simulink model "modelo_NL_con_modulador"  (R2018a)
settings: Solver=VariableStepAuto  StartTime=0.0  StopTime=30  MaxStep=1e-4  RelTol=1e-3
values from neighbouring files (symbols this model uses):
  alpha_Cu = 3.9e-3    (= 0.0039)    [proyecto_global_integrador.m]
  b_a = J_eq * n * w_pos    (= 0.0113019895361)    [proyecto_global_integrador.m]
  b_eq = b_m + b_l/r^2    (= 1.5e-05)    [proyecto_global_integrador.m]
  C_ts = 1.091    [proyecto_global_integrador.m]
  J_eq = J_m + J_l/r^2    (= 5.65099476805e-06)    [proyecto_global_integrador.m]
  k_sa = J_eq * n * w_pos^2    (= 9.04159162887)    [proyecto_global_integrador.m]
  k_sia = J_eq * w_pos^3    (= 2893.30932124)    [proyecto_global_integrador.m]
  Ke_theta = 2*polos_observador - b_eq/J_eq    (= 6397.34560009)    [proyecto_global_integrador.m]
  Ke_w = polos_observador^2 - Ke_theta * b_eq/J_eq    (= 10223018.8864)    [proyecto_global_integrador.m]
  L_d = 6.6e-3    (= 0.0066)    [proyecto_global_integrador.m]
  L_ls = 0.8e-3    (= 0.0008)    [proyecto_global_integrador.m]
  L_q = 5.8e-3    (= 0.0058)    [proyecto_global_integrador.m]
  lambda_m = 0.01546    [proyecto_global_integrador.m]
  P_p = 3    [proyecto_global_integrador.m]
  r = 314.3008    [proyecto_global_integrador.m]
  R_s = 1.02    [polos_choreo_no_se_puede_robar_mas_con_esto.m]    (also in proyecto_global_integrador.m)
  R_tsamb = 55    [proyecto_global_integrador.m]
  Rp_0 = 4    [proyecto_global_integrador.m]
  Rp_d = 33    [proyecto_global_integrador.m]
  Rp_q = 29    [proyecto_global_integrador.m]
  T_ambmax = 40    [proyecto_global_integrador.m]
libraries: simulink x4, peTransforms x2
settings Model: Creator=gabrielq  LastModifiedBy=wafle

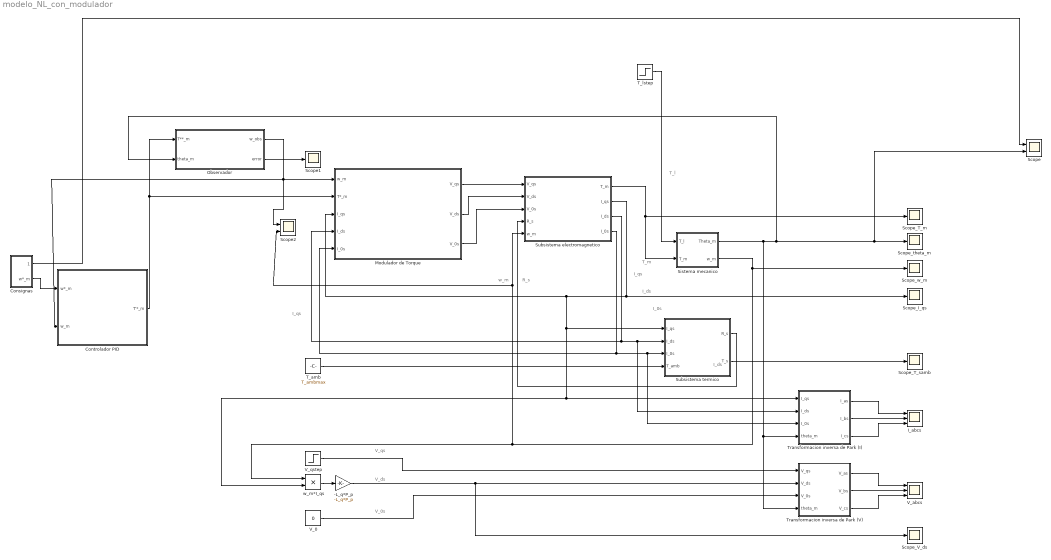
== system modelo_NL_con_modulador ==
  note: I_ds
  note: V_0s
  note: V_ds
  note: T_l
  note: V_qs
  note: T_m
  note: R_s
  note: I_0s
  note: I_ds
  note: I_qs
  note: I_qs
  note: w_m
  -L_q*P_p : Gain  Gain=-L_q*P_p
  Consignas : Subsystem
  Controlador PID : Subsystem
  I_abcs : Scope  NumInputPorts=3
  Modulador de Torque : Subsystem
  "Observador " : Subsystem
  Scope : Scope  NumInputPorts=2
  Scope1 : Scope
  Scope2 : Scope  NumInputPorts=2
  Scope_I_qs : Scope
  Scope_T_m : Scope
  Scope_T_samb : Scope
  Scope_V_ds : Scope
  Scope_theta_m : Scope
  Scope_w_m : Scope
  Sistema mecanico : Subsystem
  Subsistema electromagnetico : Subsystem
  Subsistema termico : Subsystem
  T_amb : Constant  Value=T_ambmax
  T_lstep : Step  Time=0.3  After=1.57  SampleTime=0
  Transformacion inversa de Park (I) : Subsystem
  Transformacion inversa de Park (V) : Subsystem
  V_0 : Constant  Value=0
  V_abcs : Scope  NumInputPorts=3
  V_qstep : Step  Time=0.1  After=19.596  SampleTime=0
  w_m*I_qs : Product
  wires:
  w_m*I_qs/1 -> -L_q*P_p/1
  -L_q*P_p/1 -> Scope_V_ds/1, Transformacion inversa de Park (V)/2(V_ds)
  V_qstep/1 -> Transformacion inversa de Park (V)/1(V_qs)
  V_0/1 -> Transformacion inversa de Park (V)/3(V_0s)
  Subsistema electromagnetico/2(I_qs) -> Modulador de Torque/3(I_qs), Subsistema termico/1(I_qs), w_m*I_qs/2, Transformacion inversa de Park (I)/1(I_qs), Scope_I_qs/1
  Subsistema electromagnetico/3(I_ds) -> Transformacion inversa de Park (I)/2(I_ds), Subsistema termico/2(I_ds), Modulador de Torque/4(I_ds)
  Subsistema electromagnetico/4(I_0s) -> Modulador de Torque/5(I_0s), Transformacion inversa de Park (I)/3(I_0s), Subsistema termico/3(I_0s)
  Subsistema electromagnetico/1(T_m) -> Sistema mecanico/2(T_m), Scope_T_m/1
  Sistema mecanico/2(w_m) -> Scope2/2, Subsistema electromagnetico/5(w_m), w_m*I_qs/1, Scope_w_m/1
  T_lstep/1 -> Sistema mecanico/1(T_l)
  Subsistema termico/2(T_s) -> Scope_T_samb/1
  T_amb/1 -> Subsistema termico/4(T_amb)
  Subsistema termico/1(R_s) -> Subsistema electromagnetico/4(R_s)
  Transformacion inversa de Park (I)/1(I_as) -> I_abcs/1
  Transformacion inversa de Park (I)/2(I_bs) -> I_abcs/2
  Transformacion inversa de Park (I)/3(I_cs) -> I_abcs/3
  Transformacion inversa de Park (V)/1(V_as) -> V_abcs/1
  Transformacion inversa de Park (V)/2(V_bs) -> V_abcs/2
  Transformacion inversa de Park (V)/3(V_cs) -> V_abcs/3
  "Observador "/1("w_obs ") -> Controlador PID/2(w_m), Scope2/1, Modulador de Torque/1(w_m)
  Controlador PID/1(T'*_m) -> "Observador "/1("T**_m "), Modulador de Torque/2(T*_m)
  Modulador de Torque/1(V_qs) -> Subsistema electromagnetico/1(V_qs)
  Modulador de Torque/3(V_0s) -> Subsistema electromagnetico/3(V_0s)
  Modulador de Torque/2(V_ds) -> Subsistema electromagnetico/2(V_ds)
  Consignas/2(w*_m) -> Controlador PID/1(w*_m)
  Consignas/1(theta*_m) -> Scope/1
  Sistema mecanico/1(Theta_m) -> "Observador "/2("theta_m "), Scope/2, Scope_theta_m/1, Transformacion inversa de Park (V)/4(theta_m), Transformacion inversa de Park (I)/4(theta_m)
  "Observador "/2("error ") -> Scope1/1

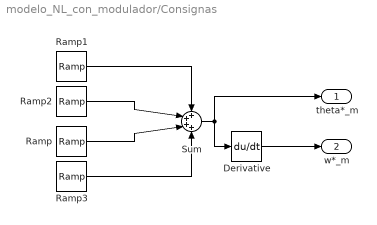
== system modelo_NL_con_modulador/Consignas ==
  Derivative : Derivative
  Ramp : simulink/Sources/Ramp  slope=-2*pi/5  start=15  InitialOutput=0
  Ramp1 : simulink/Sources/Ramp  slope=2*pi/5  start=5  InitialOutput=0
  Ramp2 : simulink/Sources/Ramp  slope=-2*pi/5  start=10  InitialOutput=0
  Ramp3 : simulink/Sources/Ramp  slope=2*pi/5  start=20  InitialOutput=0
  Sum : Sum  Inputs=4
  theta*_m : Outport
  w*_m : Outport  Port=2
  wires:
  Ramp3/1 -> Sum/4
  Ramp/1 -> Sum/3
  Derivative/1 -> w*_m/1
  Ramp2/1 -> Sum/2
  Sum/1 -> Derivative/1, theta*_m/1
  Ramp1/1 -> Sum/1

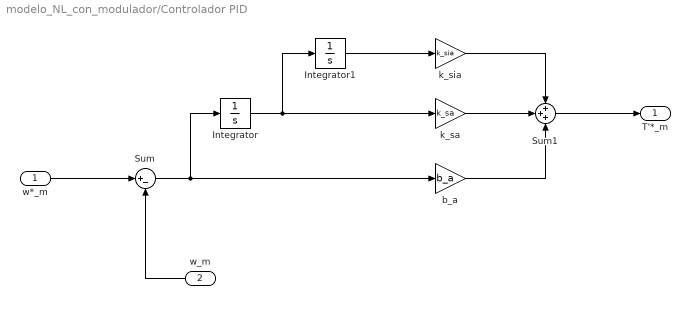
== system modelo_NL_con_modulador/Controlador PID ==
  w*_m : Inport
  w_m : Inport  Port=2
  Integrator : Integrator
  Integrator1 : Integrator
  Sum : Sum  Inputs=|+-
  Sum1 : Sum  Inputs=+++
  b_a : Gain  Gain=b_a
  k_sa : Gain  Gain=k_sa
  k_sia : Gain  Gain=k_sia
  T'*_m : Outport
  wires:
  Integrator/1 -> k_sa/1, Integrator1/1
  Sum1/1 -> T'*_m/1
  k_sa/1 -> Sum1/2
  Sum/1 -> b_a/1, Integrator/1
  w*_m/1 -> Sum/1
  k_sia/1 -> Sum1/1
  Integrator1/1 -> k_sia/1
  b_a/1 -> Sum1/3
  w_m/1 -> Sum/2

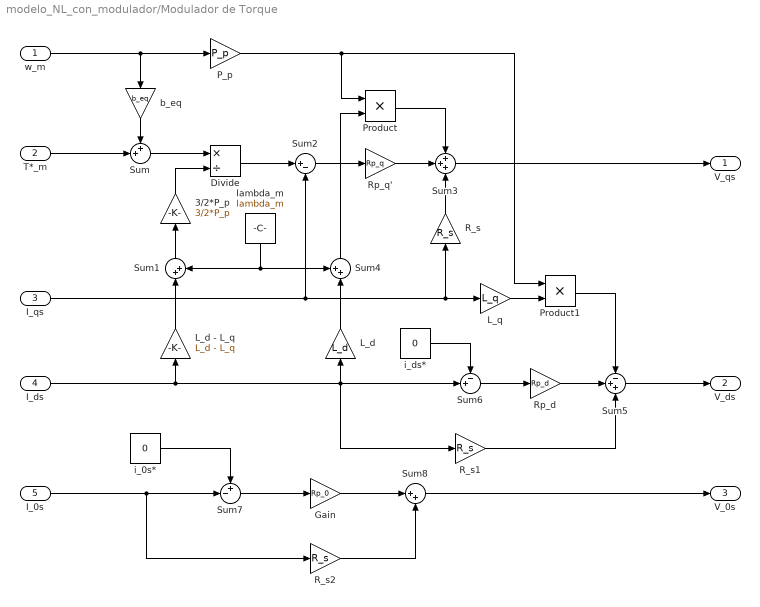
== system modelo_NL_con_modulador/Modulador de Torque ==
  w_m : Inport
  T*_m : Inport  Port=2
  I_qs : Inport  Port=3
  I_ds : Inport  Port=4
  I_0s : Inport  Port=5
  " lambda_m" : Constant  Value=lambda_m
  3/2*P_p : Gain  Gain=3/2*P_p
  Divide : Product  Inputs=*/
  Gain : Gain  Gain=Rp_0
  L_d : Gain  Gain=L_d
  L_d - L_q : Gain  Gain=L_d - L_q
  L_q : Gain  Gain=L_q
  P_p : Gain  Gain=P_p
  Product : Product
  Product1 : Product
  R_s : Gain  Gain=R_s
  R_s1 : Gain  Gain=R_s
  R_s2 : Gain  Gain=R_s
  Rp_d : Gain  Gain=Rp_d
  Rp_q' : Gain  Gain=Rp_q
  Sum : Sum  Inputs=++|
  Sum1 : Sum  Inputs=|++
  Sum2 : Sum  Inputs=|+-
  Sum3 : Sum  Inputs=+++
  Sum4 : Sum  Inputs=++|
  Sum5 : Sum  Inputs=-++
  Sum6 : Sum  Inputs=-+|
  Sum7 : Sum  Inputs=+-|
  Sum8 : Sum  Inputs=|++
  "b_eq " : Gain  Gain=b_eq
  i_0s* : Constant  Value=0
  i_ds* : Constant  Value=0
  V_qs : Outport
  V_ds : Outport  Port=2
  V_0s : Outport  Port=3
  wires:
  Sum7/1 -> Gain/1
  I_qs/1 -> R_s/1, L_q/1, Sum2/2
  R_s/1 -> Sum3/3
  Rp_q'/1 -> Sum3/2
  3/2*P_p/1 -> Divide/2
  Sum3/1 -> V_qs/1
  Sum4/1 -> Product/2
  I_ds/1 -> L_d - L_q/1, L_d/1, Sum6/2, R_s1/1
  Sum1/1 -> 3/2*P_p/1
  Divide/1 -> Sum2/1
  Sum2/1 -> Rp_q'/1
  Sum5/1 -> V_ds/1
  Sum8/1 -> V_0s/1
  L_d/1 -> Sum4/2
  Gain/1 -> Sum8/1
  i_ds*/1 -> Sum6/1
  P_p/1 -> Product/1, Product1/1
  I_0s/1 -> Sum7/2, R_s2/1
  Sum6/1 -> Rp_d/1
  L_q/1 -> Product1/2
  " lambda_m"/1 -> Sum1/2, Sum4/1
  Rp_d/1 -> Sum5/2
  "b_eq "/1 -> Sum/1
  w_m/1 -> "b_eq "/1, P_p/1
  R_s1/1 -> Sum5/3
  L_d - L_q/1 -> Sum1/1
  Sum/1 -> Divide/1
  Product/1 -> Sum3/1
  i_0s*/1 -> Sum7/1
  Product1/1 -> Sum5/1
  R_s2/1 -> Sum8/2
  T*_m/1 -> Sum/2

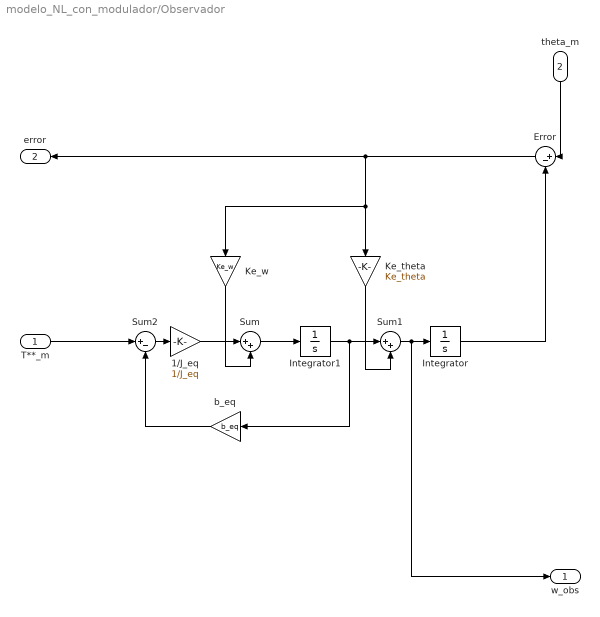
== system modelo_NL_con_modulador/Observador  ==
  "T**_m " : Inport
  "theta_m " : Inport  Port=2
  1/J_eq : Gain  Gain=1/J_eq
  "Error " : Sum  Inputs=|+-
  Integrator : Integrator
  Integrator1 : Integrator
  Ke_theta : Gain  Gain=Ke_theta
  "Ke_w " : Gain  Gain=Ke_w
  Sum : Sum  Inputs=|++
  Sum1 : Sum  Inputs=|++
  Sum2 : Sum  Inputs=|+-
  b_eq : Gain  Gain=b_eq
  "w_obs " : Outport
  "error " : Outport  Port=2
  wires:
  "Error "/1 -> "Ke_w "/1, Ke_theta/1, "error "/1
  Integrator1/1 -> b_eq/1, Sum1/1
  Sum1/1 -> "w_obs "/1, Integrator/1
  "theta_m "/1 -> "Error "/1
  Integrator/1 -> "Error "/2
  1/J_eq/1 -> Sum/1
  "Ke_w "/1 -> Sum/2
  Sum/1 -> Integrator1/1
  "T**_m "/1 -> Sum2/1
  Ke_theta/1 -> Sum1/2
  Sum2/1 -> 1/J_eq/1
  b_eq/1 -> Sum2/2

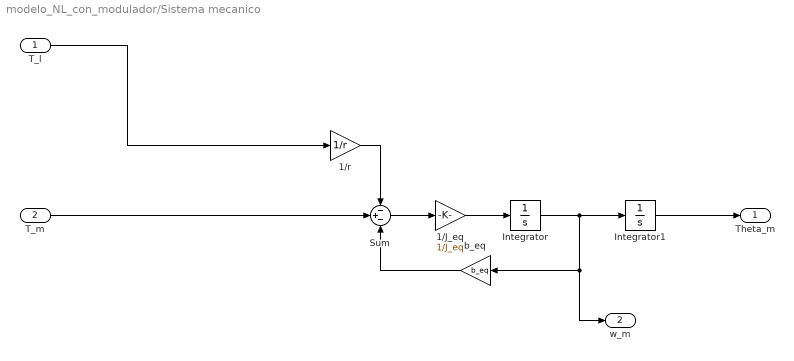
== system modelo_NL_con_modulador/Sistema mecanico ==
  T_l : Inport
  T_m : Inport  Port=2
  1/J_eq : Gain  Gain=1/J_eq
  1/r : Gain  Gain=1/r
  Integrator : Integrator
  Integrator1 : Integrator
  Sum : Sum  Inputs=-+-
  b_eq : Gain  Gain=b_eq
  Theta_m : Outport
  w_m : Outport  Port=2
  wires:
  b_eq/1 -> Sum/3
  1/J_eq/1 -> Integrator/1
  T_l/1 -> 1/r/1
  Integrator1/1 -> Theta_m/1
  Sum/1 -> 1/J_eq/1
  T_m/1 -> Sum/2
  Integrator/1 -> Integrator1/1, w_m/1, b_eq/1
  1/r/1 -> Sum/1

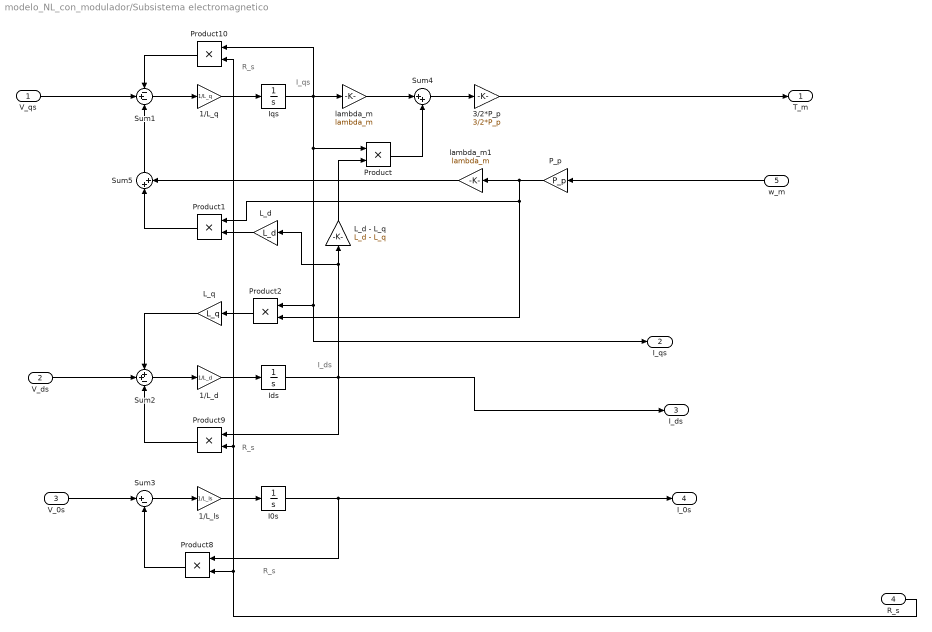
== system modelo_NL_con_modulador/Subsistema electromagnetico ==
  note: I_ds
  note: I_qs
  note: R_s
  note: R_s
  note: R_s
  V_qs : Inport
  V_ds : Inport  Port=2
  V_0s : Inport  Port=3
  R_s : Inport  Port=4
  w_m : Inport  Port=5
  1/L_d : Gain  Gain=1/L_d
  1/L_ls : Gain  Gain=1/L_ls
  1/L_q : Gain  Gain=1/L_q
  3/2*P_p : Gain  Gain=3/2*P_p
  I0s : Integrator
  Ids : Integrator
  Iqs : Integrator
  L_d : Gain  Gain=L_d
  L_d - L_q : Gain  Gain=L_d - L_q
  L_q : Gain  Gain=L_q
  P_p : Gain  Gain=P_p
  Product{,1..2,8..10} (6 alike) : Product
  Sum1 : Sum  Inputs=-+-
  Sum2 : Sum  Inputs=++-
  Sum3 : Sum  Inputs=|+-
  Sum4 : Sum  Inputs=|++
  Sum5 : Sum  Inputs=|++
  lambda_m : Gain  Gain=lambda_m
  lambda_m1 : Gain  Gain=lambda_m
  T_m : Outport
  I_qs : Outport  Port=2
  I_ds : Outport  Port=3
  I_0s : Outport  Port=4
  wires:
  Sum2/1 -> 1/L_d/1
  V_ds/1 -> Sum2/2
  I0s/1 -> I_0s/1, Product8/1
  1/L_ls/1 -> I0s/1
  L_d/1 -> Product1/2
  w_m/1 -> P_p/1
  R_s/1 -> Product10/2, Product9/2, Product8/2
  P_p/1 -> lambda_m1/1, Product2/2, Product1/1
  L_d - L_q/1 -> Product/2
  Sum5/1 -> Sum1/3
  Product8/1 -> Sum3/2
  Sum3/1 -> 1/L_ls/1
  V_0s/1 -> Sum3/1
  Ids/1 -> I_ds/1, L_d/1, L_d - L_q/1, Product9/1
  Sum1/1 -> 1/L_q/1
  Product10/1 -> Sum1/1
  Iqs/1 -> I_qs/1, Product2/1, Product/1, Product10/1, lambda_m/1
  Product/1 -> Sum4/2
  L_q/1 -> Sum2/1
  V_qs/1 -> Sum1/2
  Product1/1 -> Sum5/1
  lambda_m1/1 -> Sum5/2
  Sum4/1 -> 3/2*P_p/1
  1/L_d/1 -> Ids/1
  3/2*P_p/1 -> T_m/1
  1/L_q/1 -> Iqs/1
  Product9/1 -> Sum2/3
  lambda_m/1 -> Sum4/1
  Product2/1 -> L_q/1

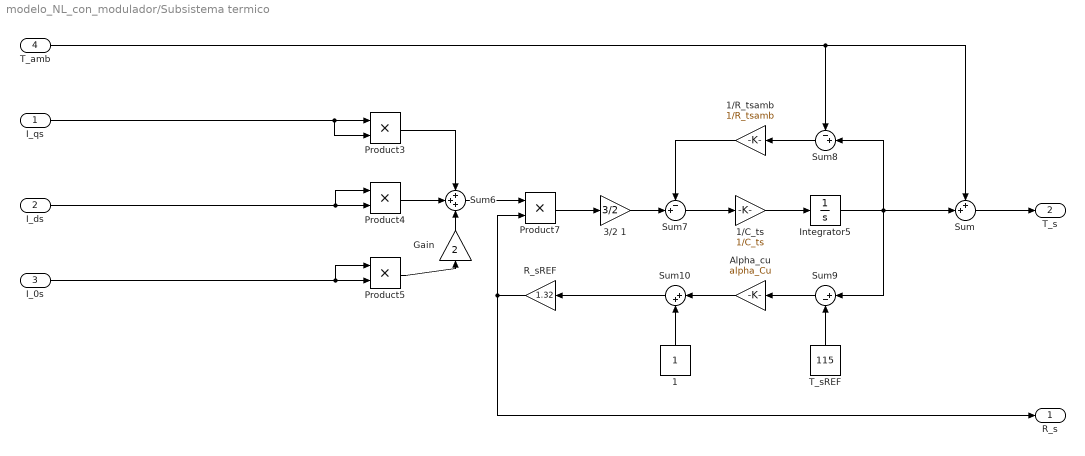
== system modelo_NL_con_modulador/Subsistema termico ==
  I_qs : Inport
  I_ds : Inport  Port=2
  I_0s : Inport  Port=3
  T_amb : Inport  Port=4
  1 : Constant
  1/C_ts : Gain  Gain=1/C_ts
  1/R_tsamb : Gain  Gain=1/R_tsamb
  3/2 1 : Gain  Gain=3/2
  Alpha_cu : Gain  Gain=alpha_Cu
  Gain : Gain  Gain=2
  Integrator5 : Integrator
  Product{3..5,7} (4 alike) : Product
  "R_sREF " : Gain  Gain=1.32
  Sum : Sum  Inputs=++|
  Sum10 : Sum  Inputs=|++
  Sum6 : Sum  Inputs=+++
  Sum7 : Sum  Inputs=-+|
  Sum8 : Sum  Inputs=-+|
  Sum9 : Sum  Inputs=|+-
  T_sREF : Constant  Value=115
  R_s : Outport
  T_s : Outport  Port=2
  wires:
  Product4/1 -> Sum6/2
  Product3/1 -> Sum6/1
  1/R_tsamb/1 -> Sum7/1
  Sum6/1 -> Product7/1
  Sum8/1 -> 1/R_tsamb/1
  I_ds/1 -> Product4/2, Product4/1
  Sum7/1 -> 1/C_ts/1
  Product7/1 -> 3/2 1/1
  I_qs/1 -> Product3/2, Product3/1
  I_0s/1 -> Product5/1, Product5/2
  Gain/1 -> Sum6/3
  T_amb/1 -> Sum/1, Sum8/1
  Sum9/1 -> Alpha_cu/1
  Sum10/1 -> "R_sREF "/1
  1/C_ts/1 -> Integrator5/1
  Product5/1 -> Gain/1
  Alpha_cu/1 -> Sum10/1
  "R_sREF "/1 -> Product7/2, R_s/1
  Integrator5/1 -> Sum/2, Sum9/1, Sum8/2
  3/2 1/1 -> Sum7/2
  T_sREF/1 -> Sum9/2
  1/1 -> Sum10/2
  Sum/1 -> T_s/1

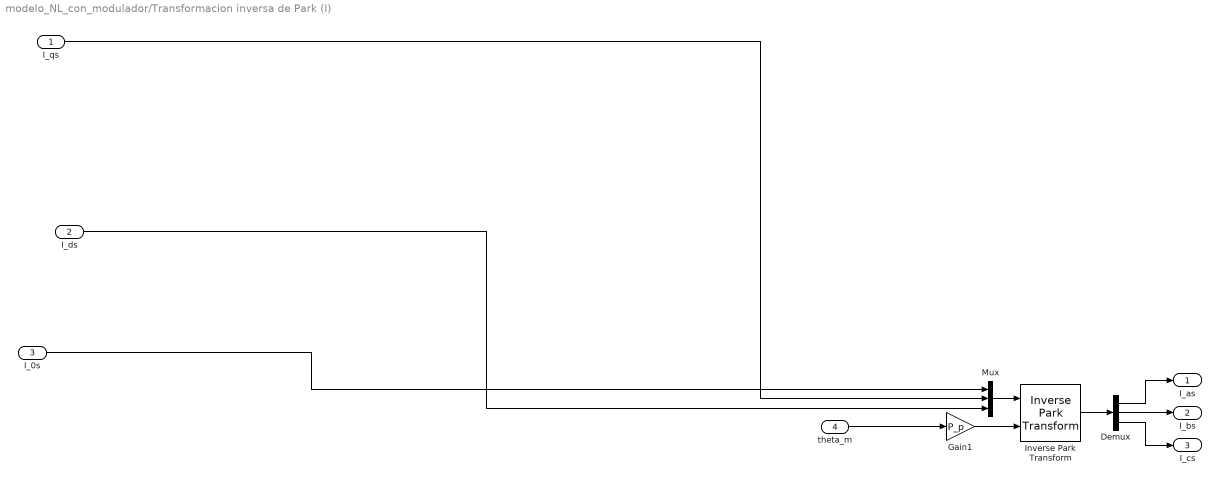
== system modelo_NL_con_modulador/Transformacion inversa de Park (I) ==
  I_qs : Inport
  I_ds : Inport  Port=2
  I_0s : Inport  Port=3
  theta_m : Inport  Port=4
  Demux : Demux  Outputs=3
  Gain1 : Gain  Gain=P_p
  Inverse Park Transform : peTransforms/Inverse Park Transform  AxisAlignment=Q-axis  PowerInvariant=off
  Mux : Mux  Inputs=3
  I_as : Outport
  I_bs : Outport  Port=2
  I_cs : Outport  Port=3
  wires:
  I_qs/1 -> Mux/2
  Mux/1 -> Inverse Park Transform/1
  Gain1/1 -> Inverse Park Transform/2
  Inverse Park Transform/1 -> Demux/1
  theta_m/1 -> Gain1/1
  I_ds/1 -> Mux/3
  Demux/2 -> I_bs/1
  Demux/1 -> I_as/1
  Demux/3 -> I_cs/1
  I_0s/1 -> Mux/1

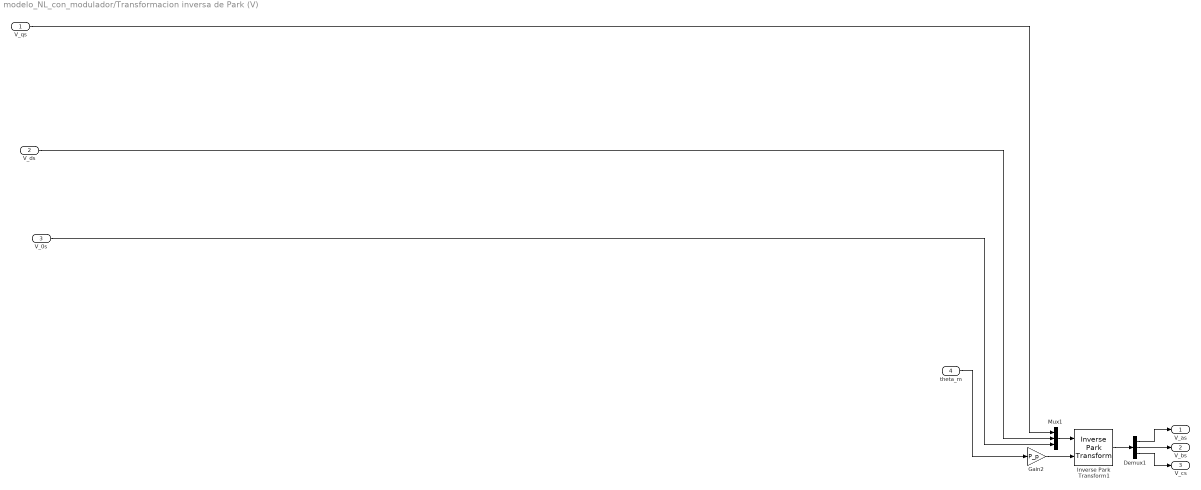
== system modelo_NL_con_modulador/Transformacion inversa de Park (V) ==
  V_qs : Inport
  V_ds : Inport  Port=2
  V_0s : Inport  Port=3
  theta_m : Inport  Port=4
  Demux1 : Demux  Outputs=3
  Gain2 : Gain  Gain=P_p
  Inverse Park Transform1 : peTransforms/Inverse Park Transform  AxisAlignment=Q-axis  PowerInvariant=off
  Mux1 : Mux  Inputs=3
  V_as : Outport
  V_bs : Outport  Port=2
  V_cs : Outport  Port=3
  wires:
  theta_m/1 -> Gain2/1
  Gain2/1 -> Inverse Park Transform1/2
  V_ds/1 -> Mux1/2
  V_qs/1 -> Mux1/1
  Inverse Park Transform1/1 -> Demux1/1
  Demux1/3 -> V_cs/1
  Demux1/2 -> V_bs/1
  Mux1/1 -> Inverse Park Transform1/1
  V_0s/1 -> Mux1/3
  Demux1/1 -> V_as/1
